simulink library "VIRTTAC_Castor"  (Simulink 7.0)
settings Model: Creator=deil_ch  LastModifiedBy=feza_ni

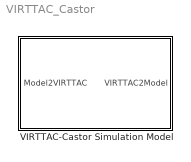
== system VIRTTAC_Castor ==
  VIRTTAC-Castor Simulation Model : Subsystem
      mask Type: VIRTTAC-Castor Simulation
      mask Description: The block contains the simulation of VIRTTAC-Castor and shall not be modified by any user!
      mask Display: image(get_param(gcbh,'UserData'));

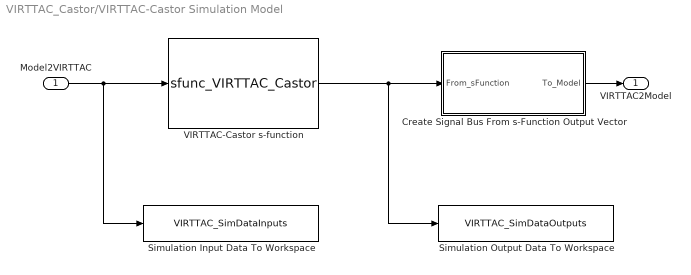
== system VIRTTAC_Castor/VIRTTAC-Castor Simulation Model ==
  Model2VIRTTAC : Inport  PortDimensions=VIRTTAC.Sim.InputPortDim  DataType=double
  Create Signal Bus From s-Function Output Vector : Subsystem
  Simulation Input Data To Workspace : ToWorkspace  VariableName=VIRTTAC_SimDataInputs  SampleTime=-1  SaveFormat=Structure With Time
  Simulation Output Data To Workspace : ToWorkspace  VariableName=VIRTTAC_SimDataOutputs  SampleTime=-1  SaveFormat=Structure With Time
  VIRTTAC-Castor s-function : S-Function  FunctionName=sfunc_VIRTTAC_Castor  Parameters=VIRTTAC.Sim.SampleTime, VIRTTAC.Sim.Trimming
      mask Display: image(get_param(gcbh,'UserData'));
  VIRTTAC2Model : Outport
  wires:
  VIRTTAC-Castor s-function/1 -> Simulation Output Data To Workspace/1, Create Signal Bus From s-Function Output Vector/1(From_sFunction)
  Model2VIRTTAC/1 -> VIRTTAC-Castor s-function/1, Simulation Input Data To Workspace/1
  Create Signal Bus From s-Function Output Vector/1(To_Model) -> VIRTTAC2Model/1

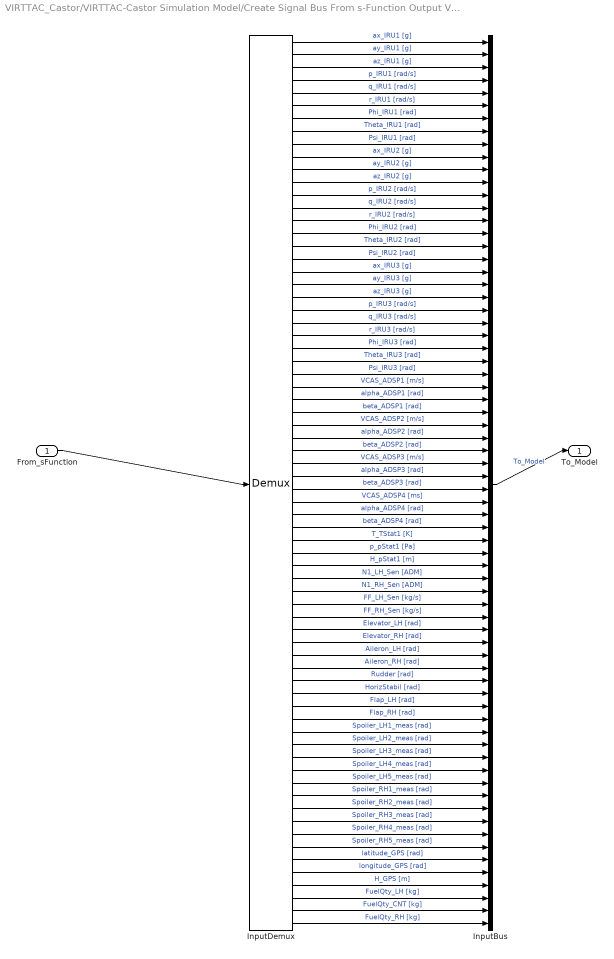
== system VIRTTAC_Castor/VIRTTAC-Castor Simulation Model/Create Signal Bus From s-Function Output Vector ==
  From_sFunction : Inport  PortDimensions=70  DataType=double
  InputBus : BusCreator  Inputs=70
  InputDemux : Demux  Outputs=70
  To_Model : Outport
  wires:
  From_sFunction/1 -> InputDemux/1
  InputBus/1 -> To_Model/1  "To_Model"
  InputDemux/1 -> InputBus/1  "ax_IRU1 [g]"
  InputDemux/2 -> InputBus/2  "ay_IRU1 [g]"
  InputDemux/3 -> InputBus/3  "az_IRU1 [g]"
  InputDemux/4 -> InputBus/4  "p_IRU1 [rad/s]"
  InputDemux/5 -> InputBus/5  "q_IRU1 [rad/s]"
  InputDemux/6 -> InputBus/6  "r_IRU1 [rad/s]"
  InputDemux/7 -> InputBus/7  "Phi_IRU1 [rad]"
  InputDemux/8 -> InputBus/8  "Theta_IRU1 [rad]"
  InputDemux/9 -> InputBus/9  "Psi_IRU1 [rad]"
  InputDemux/10 -> InputBus/10  "ax_IRU2 [g]"
  InputDemux/11 -> InputBus/11  "ay_IRU2 [g]"
  InputDemux/12 -> InputBus/12  "az_IRU2 [g]"
  InputDemux/13 -> InputBus/13  "p_IRU2 [rad/s]"
  InputDemux/14 -> InputBus/14  "q_IRU2 [rad/s]"
  InputDemux/15 -> InputBus/15  "r_IRU2 [rad/s]"
  InputDemux/16 -> InputBus/16  "Phi_IRU2 [rad]"
  InputDemux/17 -> InputBus/17  "Theta_IRU2 [rad]"
  InputDemux/18 -> InputBus/18  "Psi_IRU2 [rad]"
  InputDemux/19 -> InputBus/19  "ax_IRU3 [g]"
  InputDemux/20 -> InputBus/20  "ay_IRU3 [g]"
  InputDemux/21 -> InputBus/21  "az_IRU3 [g]"
  InputDemux/22 -> InputBus/22  "p_IRU3 [rad/s]"
  InputDemux/23 -> InputBus/23  "q_IRU3 [rad/s]"
  InputDemux/24 -> InputBus/24  "r_IRU3 [rad/s]"
  InputDemux/25 -> InputBus/25  "Phi_IRU3 [rad]"
  InputDemux/26 -> InputBus/26  "Theta_IRU3 [rad]"
  InputDemux/27 -> InputBus/27  "Psi_IRU3 [rad]"
  InputDemux/28 -> InputBus/28  "VCAS_ADSP1 [m/s]"
  InputDemux/29 -> InputBus/29  "alpha_ADSP1 [rad]"
  InputDemux/30 -> InputBus/30  "beta_ADSP1 [rad]"
  InputDemux/31 -> InputBus/31  "VCAS_ADSP2 [m/s]"
  InputDemux/32 -> InputBus/32  "alpha_ADSP2 [rad]"
  InputDemux/33 -> InputBus/33  "beta_ADSP2 [rad]"
  InputDemux/34 -> InputBus/34  "VCAS_ADSP3 [m/s]"
  InputDemux/35 -> InputBus/35  "alpha_ADSP3 [rad]"
  InputDemux/36 -> InputBus/36  "beta_ADSP3 [rad]"
  InputDemux/37 -> InputBus/37  "VCAS_ADSP4 [ms]"
  InputDemux/38 -> InputBus/38  "alpha_ADSP4 [rad]"
  InputDemux/39 -> InputBus/39  "beta_ADSP4 [rad]"
  InputDemux/40 -> InputBus/40  "T_TStat1 [K]"
  InputDemux/41 -> InputBus/41  "p_pStat1 [Pa]"
  InputDemux/42 -> InputBus/42  "H_pStat1 [m]"
  InputDemux/43 -> InputBus/43  "N1_LH_Sen [ADM]"
  InputDemux/44 -> InputBus/44  "N1_RH_Sen [ADM]"
  InputDemux/45 -> InputBus/45  "FF_LH_Sen [kg/s]"
  InputDemux/46 -> InputBus/46  "FF_RH_Sen [kg/s]"
  InputDemux/47 -> InputBus/47  "Elevator_LH [rad]"
  InputDemux/48 -> InputBus/48  "Elevator_RH [rad]"
  InputDemux/49 -> InputBus/49  "Aileron_LH [rad]"
  InputDemux/50 -> InputBus/50  "Aileron_RH [rad]"
  InputDemux/51 -> InputBus/51  "Rudder [rad]"
  InputDemux/52 -> InputBus/52  "HorizStabil [rad]"
  InputDemux/53 -> InputBus/53  "Flap_LH [rad]"
  InputDemux/54 -> InputBus/54  "Flap_RH [rad]"
  InputDemux/55 -> InputBus/55  "Spoiler_LH1_meas [rad]"
  InputDemux/56 -> InputBus/56  "Spoiler_LH2_meas [rad]"
  InputDemux/57 -> InputBus/57  "Spoiler_LH3_meas [rad]"
  InputDemux/58 -> InputBus/58  "Spoiler_LH4_meas [rad]"
  InputDemux/59 -> InputBus/59  "Spoiler_LH5_meas [rad]"
  InputDemux/60 -> InputBus/60  "Spoiler_RH1_meas [rad]"
  InputDemux/61 -> InputBus/61  "Spoiler_RH2_meas [rad]"
  InputDemux/62 -> InputBus/62  "Spoiler_RH3_meas [rad]"
  InputDemux/63 -> InputBus/63  "Spoiler_RH4_meas [rad]"
  InputDemux/64 -> InputBus/64  "Spoiler_RH5_meas [rad]"
  InputDemux/65 -> InputBus/65  "latitude_GPS [rad]"
  InputDemux/66 -> InputBus/66  "longitude_GPS [rad]"
  InputDemux/67 -> InputBus/67  "H_GPS [m]"
  InputDemux/68 -> InputBus/68  "FuelQty_LH [kg]"
  InputDemux/69 -> InputBus/69  "FuelQty_CNT [kg]"
  InputDemux/70 -> InputBus/70  "FuelQty_RH [kg]"
